simulink model "UNIFIER"  (R2023b)
settings: Solver=ode1  StartTime=0.0  StopTime=194  FixedStep=1/500  RelTol=1e-3
values from neighbouring files (symbols this model uses):
  b = 20.11467    [UNIFIERLanding_20240613_190735.mat]    (also in UNIFIER_LOAD.m; UNIFIER_LOADsim.m; UNIFIER_trim_out_20240612_032607.mat)
  c = 1.43676    [UNIFIERLanding_20240613_190735.mat]    (also in UNIFIER_LOAD.m; UNIFIER_LOADsim.m; UNIFIER_trim_out_20240612_032607.mat)
  DEP_INTEG_IC = 117.49388    [UNIFIER_LOAD.m]    (also in UNIFIER_LOADsim.m; UNIFIER_trim_out_20240612_032607.mat)
  dp_DEP =     [UNIFIERLanding_20240613_190735.mat]    (also in UNIFIER_trim_out_20240612_032607.mat)
  dp_FUSE_FIN =     [UNIFIER_trim_out_20240612_032607.mat]
  dp_HTU =     [UNIFIERLanding_20240613_190735.mat]    (also in UNIFIER_trim_out_20240612_032607.mat)
  dp_VTAIL =     [UNIFIER_trim_out_20240612_032607.mat]
  dp_VTAIL_INDUCED =     [UNIFIER_trim_out_20240612_032607.mat]
  dp_WING_root =     [UNIFIER_trim_out_20240612_032607.mat]
  dp_WING_tip =     [UNIFIER_trim_out_20240612_032607.mat]
  dumax = [1.0471975512 1.0471975512 1.0471975512 0.174532925199 2 2 2]    [UNIFIERLanding_20240613_190735.mat]
  Euler0 = xstar(7:9)'    [UNIFIER_6DOFsim_init.m]    (also in UNIFIER_LOAD.m = [0, 0, 0]; UNIFIER_LOADsim.m = [0, 0, 0]; UNIFIER_trim_out_20240612_032607.mat = [3.43106170069e-06 0.0515008506278 -2.79252663434])
  ground_alt = 0    [UNIFIER_LOAD.m]    (also in UNIFIER_LOADsim.m; UNIFIER_trim_out_20240612_032607.mat)
  m = 7057    [UNIFIERLanding_20240613_190735.mat]    (also in UNIFIER_LOAD.m; UNIFIER_LOADsim.m; UNIFIER_trim_out_20240612_032607.mat)
  omegab0 = xstar(10:12)'    [UNIFIER_6DOFsim_init.m]    (also in UNIFIER_LOAD.m = [0,0,0]; UNIFIER_LOADsim.m = [0,0,0]; UNIFIER_trim_out_20240612_032607.mat = [0 0 0])
  S = 29.98388    [UNIFIERLanding_20240613_190735.mat]    (also in UNIFIER_LOAD.m; UNIFIER_LOADsim.m; UNIFIER_trim_out_20240612_032607.mat)
  sensor_delay_steps = 5    [UNIFIER_LOAD.m]    (also in UNIFIER_LOADsim.m; UNIFIER_trim_out_20240612_032607.mat)
  solution =     [UNIFIERLanding_20240613_190735.mat]
  u1_0 = [ustar(1), -1*ustar(1), ustar(3)-ustar(2), ustar(3)+ustar(2), ustar(4), ustar(4)]    [UNIFIER_6DOFsim_init.m]    (also in UNIFIER_LOAD.m = [2.1112539e-05, -2.1112539e-05, -0.085004635, -0.084972650, ; UNIFIER_LOADsim.m = [2.1112539e-05, -2.1112539e-05, -0.085004635, -0.084972650, ; UNIFIER_trim_out_20240612_032607.mat = [2.1112539e-05 -2.1112539e-05 -0.085004635 -0.08497265 0.197)
  u2_0 = ones(1,12) .* ustar(5)    [UNIFIER_6DOFsim_init.m]    (also in UNIFIER_LOAD.m = ones(1,12) .* 0.4252; UNIFIER_LOADsim.m = ones(1,12) .* 0.4252; UNIFIER_trim_out_20240612_032607.mat = [0.4252 0.4252 0.4252 0.4252 0.4252 0.4252 0.4252 0.4252 0.4)
  u3_0 = ustar(7)    [UNIFIER_6DOFsim_init.m]    (also in UNIFIER_LOAD.m = 0.089689; UNIFIER_LOADsim.m = 0.089689; UNIFIER_trim_out_20240612_032607.mat = 0.089689)
  u4_0 = 0    [UNIFIER_6DOFsim_init.m]    (also in UNIFIER_LOAD.m; UNIFIER_LOADsim.m; UNIFIER_trim_out_20240612_032607.mat)
  u_trim = ustar    [UNIFIER_6DOFsim_init.m]    (also in UNIFIER_LOAD.m = [0.0; UNIFIER_LOADsim.m = [0.0)
  umax = [0.436332312999 0.523598775598 0.523598775598 0.436332312999 1 1 1]    [UNIFIERLanding_20240613_190735.mat]    (also in UNIFIER_trim_out_20240612_032607.mat)
  umin = [-0.436332312999 -0.523598775598 -0.523598775598 0 0 -1 -0.5]    [UNIFIERLanding_20240613_190735.mat]    (also in UNIFIER_trim_out_20240612_032607.mat)
  Va = [72.7399985115 72.2978466179 70.3592089076 68.5755686022 67.5674222915 66.8967003826 65.8958642605 64.4243196248 62.667507398 61.0171213882 59.8601734245 59.2796795419 ... (250 elements, 250x1)]    [UNIFIERLanding_20240613_190735.mat]
  Vb0 = xstar(4:6)'    [UNIFIER_6DOFsim_init.m]    (also in UNIFIER_LOAD.m = [72.731047032614440, 0, 1.142307104518741]; UNIFIER_LOADsim.m = [72.731047032614440, 0, 1.142307104518741]; UNIFIER_trim_out_20240612_032607.mat = [52.6789583502 0 2.71559652634])
  vtail_dist_to_wing = 7.8070    (= 7.807)    [UNIFIER_LOAD.m]    (also in UNIFIER_LOADsim.m; UNIFIER_trim_out_20240612_032607.mat)
  vtail_nodes = [dp_VTAIL.Xs_LE;     dp_VTAIL.Ys_LE;     dp_VTAIL.Zs_LE]    [UNIFIER_LOAD.m]    (also in UNIFIER_LOADsim.m; UNIFIER_trim_out_20240612_032607.mat = [-16.4894695282 -2.83441376686 -2.73765826225 -16.1370849609)
  wing_nodes = [fliplr(dp_WING_tip.LE_Xs),fliplr(dp_WING_root.LE_Xs),dp_WING_root.LE_Xs,dp_WING_tip.LE_Xs;     fliplr(-dp_WING_tip.LE_Ys),fliplr(-dp_WING_root.LE_Ys),dp_WING_root.LE_Ys,dp_WING_tip.LE_Ys;     fliplr(dp_WING_tip.LE_Zs),fliplr(dp_WING_root.LE_Zs),dp_WING_root.LE_Zs,dp_WING_tip.LE_Zs]    [UNIFIER_LOAD.m]    (also in UNIFIER_LOADsim.m; UNIFIER_trim_out_20240612_032607.mat = [-7.70795631409 -9.67500019073 -0.98178178072 -7.66801691055)
  Xe0 = xstar(1:3)'    [UNIFIER_6DOFsim_init.m]    (also in UNIFIER_LOAD.m = [0,0,-1219]; UNIFIER_LOADsim.m = [0,0,-1219]; UNIFIER_trim_out_20240612_032607.mat = [0 0 -1100])
  xyz_cg = [-8.09 0 -0.2]    [UNIFIERLanding_20240613_190735.mat]    (also in UNIFIER_LOAD.m = [-8.09,0,-0.2]; UNIFIER_LOADsim.m = [-8.09,0,-0.2]; UNIFIER_trim_out_20240612_032607.mat)
  xyz_DEP = [-6.9629998 -10.05 -0.90899998 -6.921 -8.4499998 -0.792 -6.8660002 -6.8499999 -0.82300001 -6.8099999 -5.25 -0.85000002 ... (36 elements, 3x12)]    [UNIFIERLanding_20240613_190735.mat]    (also in UNIFIER_LOAD.m = [ -6.9629998	-6.9210000	-6.8660002	-6.8099999	-6.7540002	-6.; UNIFIER_LOADsim.m = [ -6.9629998	-6.9210000	-6.8660002	-6.8099999	-6.7540002	-6.; UNIFIER_trim_out_20240612_032607.mat)
undefined symbols (not defined in the file or in its folder): Earth, F, MIL, WGS84
libraries: simulink_extras x23, aerolibactuator x16, dspnetwork x15, sharedutil x14, sharedtransform x7, aerolibtransform2 x5, slpidlib x5, simulink x5, aerolibwind2 x4, matrix_library x1, shared6dof x1, aerolibatmos2 x1
(part 3 of 6)

== system UNIFIER/C7A_HARW/Aero/additionalDrag ==
  note: Landing gear drag:
      | Loftin Jr, L. K. (1980). Subsonic aircraft: Evolution and the matching of size to performance (No. L-13367).
  note: Wing mounted nacelles:
      | (Estimate using OpenVSP - Jenkinson Wing Mounted Nacelle)
      | =6*0.00043=0.00258
      | + cooling drag of 0.015
  alpha (rad) : Inport
  beta (rad) : Inport  Port=2
  Vrw_mag : Inport  Port=3
  rho (kg/m^3) : Inport  Port=4
  u4 (gear) : Inport  Port=5
  Cast : DataTypeConversion  OutDataTypeStr=single  SaturateOnIntegerOverflow=off  RndMeth=Floor
  Cast1 : DataTypeConversion  OutDataTypeStr=single  SaturateOnIntegerOverflow=off  RndMeth=Floor
  Cast2 : DataTypeConversion  OutDataTypeStr=double  SaturateOnIntegerOverflow=off  RndMeth=Floor
  Constant1 : Constant  Value=0  OutDataTypeStr=single
  Direction Cosine Matrix Body to Wind : aerolibtransform2/Direction Cosine Matrix Body to Wind
  Gain : Gain  Gain=S/2
  Math Function : Math  Operator=square
  Mux : Mux  Inputs=2
  Mux1 : Mux  Inputs=3
  Product : Product  OutDataTypeStr=single
  Product1 : Product  Multiplication=Matrix(*)
  Product2 : Product
  Product3 : Product
  Sum : Sum  Inputs=|++
  Transpose : Math  Operator=transpose
  Unary Minus : UnaryMinus
  extra_drag : Constant  Value=0.00258+0.015  OutDataTypeStr=single
  gear_drag : Constant  Value=0.015  OutDataTypeStr=single
  F_additional : Outport
  wires:
  alpha (rad)/1 -> Mux/1
  Math Function/1 -> Product/2
  Product/1 -> Unary Minus/1
  Gain/1 -> Product/1
  Product2/1 -> Gain/1
  extra_drag/1 -> Sum/1
  Vrw_mag/1 -> Math Function/1
  rho (kg/m^3)/1 -> Product2/2
  Direction Cosine Matrix Body to Wind/1 -> Cast1/1
  Mux/1 -> Cast2/1
  beta (rad)/1 -> Mux/2
  Unary Minus/1 -> Mux1/1
  Transpose/1 -> Product1/1
  Mux1/1 -> Product1/2
  Constant1/1 -> Mux1/2, Mux1/3
  Product1/1 -> Cast/1
  Cast/1 -> F_additional/1
  Cast1/1 -> Transpose/1
  Cast2/1 -> Direction Cosine Matrix Body to Wind/1
  u4 (gear)/1 -> Product3/2
  gear_drag/1 -> Product3/1
  Sum/1 -> Product2/1
  Product3/1 -> Sum/2

== system UNIFIER/C7A_HARW/EOMandEnviroment1/Conversion ==
  Vrw : Inport
  rho : Inport  Port=2
  Add : Sum
  Constant1 : Constant  Value=eps
  Demux3 : Demux  Outputs=3
  Divide1 : Product  Inputs=*/
  Dot Product : DotProduct  OutDataTypeStr=Inherit: Inherit via internal rule
  Gain : Gain  Gain=1/1.225
  Product : Product
  Sqrt : Sqrt
  Sqrt1 : Sqrt
  Trigonometric Function : Trigonometry  Operator=atan2
  Trigonometric Function1 : Trigonometry  Operator=asin
  Vrw_mag : Outport
  Vrw_mag_eas : Outport  Port=2
  alpha : Outport  Port=3
  beta : Outport  Port=4
  wires:
  Demux3/2 -> Divide1/1
  Constant1/1 -> Add/2
  Sqrt/1 -> Add/1
  Divide1/1 -> Trigonometric Function1/1
  Vrw/1 -> Dot Product/1, Dot Product/2, Demux3/1  "V_w"
  Demux3/3 -> Trigonometric Function/1
  Dot Product/1 -> Sqrt/1
  Demux3/1 -> Trigonometric Function/2
  Trigonometric Function1/1 -> beta/1  "beta"
  Trigonometric Function/1 -> alpha/1  "alpha"
  rho/1 -> Gain/1
  Gain/1 -> Sqrt1/1
  Sqrt1/1 -> Product/2
  Product/1 -> Vrw_mag_eas/1
  Add/1 -> Vrw_mag/1, Product/1, Divide1/2

== system UNIFIER/C7A_HARW/EOMandEnviroment1/Enviroment ==
  Xe : Inport
  Vb : Inport  Port=2  PortDimensions=3
  DCM : Inport  Port=3
  omega : Inport  Port=4
  Cast : DataTypeConversion  OutDataTypeStr=single  SaturateOnIntegerOverflow=off  RndMeth=Floor
  Demux : Demux  Outputs=3
  ISA Atmosphere Model : aerolibatmos2/ISA Atmosphere Model  useExtended=off  action=Warning  custom=off  viscosityOut=off  g=9.80665  gamma=1.4  R=287.0531  L=0.0065  h_trop=11000  h_strat=20000  rho0=1.225  P0=101325  T0=288.15  h0=0
  Manual Switch : ManualSwitch
  Manual Switch1 : ManualSwitch  CurrentSetting=0
  Square : Math  Operator=square
  Square Root : Sqrt
  Sum : Sum  Inputs=|++
  Sum of Elements : Sum  Inputs=+
  Sum1 : Sum  Inputs=++|
  Terminator : Terminator
  Terminator1 : Terminator
  Terminator2 : Terminator
  Unary Minus : UnaryMinus
  Wind model : Subsystem
  scope_V : Subsystem
  scope_omega : Subsystem
  Vrw : Outport
  omegaw : Outport  Port=2
  T : Outport  Port=3
  P : Outport  Port=4
  rho : Outport  Port=5
  wires:
  Xe/1 -> Demux/1
  Demux/3 -> Unary Minus/1  "z"
  Demux/1 -> Terminator/1
  Demux/2 -> Terminator1/1
  ISA Atmosphere Model/2 -> Terminator2/1
  Manual Switch/1 -> Vrw/1
  Manual Switch1/1 -> omegaw/1
  Square Root/1 -> Wind model/2(Vb_mag)
  omega/1 -> scope_omega/2(<omega>), Manual Switch1/2, Sum/2
  Wind model/2(omegab_wind) -> Sum/1
  Wind model/1(Vb_wind) -> Sum1/2
  Sum1/1 -> Manual Switch/2, scope_V/1(V_w)
  Sum/1 -> scope_omega/1(omega_w), Manual Switch1/1
  ISA Atmosphere Model/1 -> T/1  "T"
  ISA Atmosphere Model/3 -> P/1  "P"
  ISA Atmosphere Model/4 -> rho/1  "rho"
  Unary Minus/1 -> Cast/1, Wind model/1(h)  "h"
  Cast/1 -> ISA Atmosphere Model/1
  DCM/1 -> Wind model/3(DCM)
  Vb/1 -> scope_V/2(<V_b>), Manual Switch/1, Sum1/1, Square/1
  Square/1 -> Sum of Elements/1
  Sum of Elements/1 -> Square Root/1

== system UNIFIER/C7A_HARW/Subsystems/Actuators ==
  u1 : Inport
  Demux : Demux  Commented=on  Outputs=6
  Mux : Mux  Commented=on  Inputs=6
  Nonlinear Second-Order Actuator : aerolibactuator/Nonlinear Second-Order Actuator  Commented=on  wn_fin=50  z_fin=0.8  fin_max=30*pi/180  fin_min=-30*pi/180  fin_maxrate=120*pi/180  fin_act_0=0  fin_act_vel=0
  Nonlinear Second-Order Actuator1 : aerolibactuator/Nonlinear Second-Order Actuator  Commented=on  wn_fin=50  z_fin=0.8  fin_max=30*pi/180  fin_min=-30*pi/180  fin_maxrate=120*pi/180  fin_act_0=0  fin_act_vel=0
  Nonlinear Second-Order Actuator2 : aerolibactuator/Nonlinear Second-Order Actuator  Commented=on  wn_fin=50  z_fin=0.8  fin_max=25*pi/180  fin_min=0  fin_maxrate=60*pi/180  fin_act_0=0  fin_act_vel=0
  Nonlinear Second-Order Actuator3 : aerolibactuator/Nonlinear Second-Order Actuator  Commented=on  wn_fin=50  z_fin=0.8  fin_max=25*pi/180  fin_min=0  fin_maxrate=60*pi/180  fin_act_0=0  fin_act_vel=0
  Nonlinear Second-Order Actuator4 : aerolibactuator/Nonlinear Second-Order Actuator  Commented=on  wn_fin=50  z_fin=0.8  fin_max=25*pi/180  fin_min=-25*pi/180  fin_maxrate=120*pi/180  fin_act_0=0  fin_act_vel=0
  Nonlinear Second-Order Actuator5 : aerolibactuator/Nonlinear Second-Order Actuator  Commented=on  wn_fin=50  z_fin=0.8  fin_max=25*pi/180  fin_min=-25*pi/180  fin_maxrate=120*pi/180  fin_act_0=0  fin_act_vel=0
  u1_actual : Outport
  wires:
  u1/1 -> u1_actual/1
  Demux/3 -> Nonlinear Second-Order Actuator/1
  Nonlinear Second-Order Actuator/1 -> Mux/3
  Demux/4 -> Nonlinear Second-Order Actuator1/1
  Nonlinear Second-Order Actuator1/1 -> Mux/4
  Demux/5 -> Nonlinear Second-Order Actuator2/1
  Demux/6 -> Nonlinear Second-Order Actuator3/1
  Nonlinear Second-Order Actuator3/1 -> Mux/6
  Nonlinear Second-Order Actuator2/1 -> Mux/5
  Demux/1 -> Nonlinear Second-Order Actuator5/1
  Nonlinear Second-Order Actuator5/1 -> Mux/1
  Nonlinear Second-Order Actuator4/1 -> Mux/2
  Demux/2 -> Nonlinear Second-Order Actuator4/1

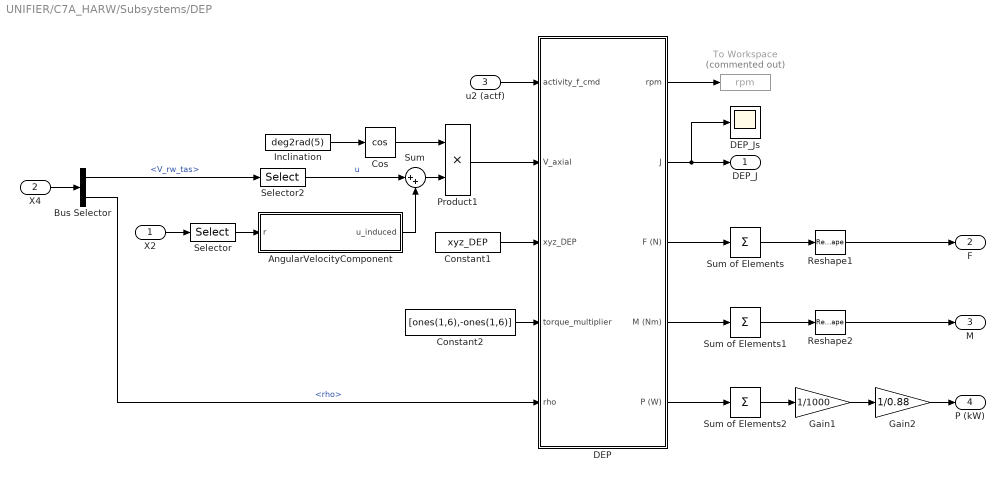
== system UNIFIER/C7A_HARW/Subsystems/DEP ==
  X2 : Inport
  X4 : Inport  Port=2
  u2 (actf) : Inport  Port=3
  AngularVelocityComponent : Subsystem
  Bus Selector : BusSelector  OutputSignals=V_rw_tas,rho
  Constant1 : Constant  Value=xyz_DEP
  Constant2 : Constant  Value=[ones(1,6),-ones(1,6)]
  Cos : Trigonometry  Operator=cos
  DEP : Subsystem  TreatAsAtomicUnit=on
  DEP_Js : Scope
  Gain1 : Gain  Gain=1/1000
  Gain2 : Gain  Gain=1/0.88
  Inclination : Constant  Value=deg2rad(5)
  Product1 : Product
  Reshape1 : Reshape
  Reshape2 : Reshape
  Selector : Selector  InputPortWidth=6  IndexOptions=Index vector (dialog)  Indices=6  OutputSizes=1
  Selector2 : Selector  InputPortWidth=3  IndexOptions=Index vector (dialog)  Indices=1  OutputSizes=1
  Sum : Sum  Inputs=|++
  Sum of Elements : Sum  Inputs=+  CollapseMode=Specified dimension  CollapseDim=2
  Sum of Elements1 : Sum  Inputs=+  CollapseMode=Specified dimension  CollapseDim=2
  Sum of Elements2 : Sum  Inputs=+  CollapseMode=Specified dimension
  To Workspace : ToWorkspace  Commented=on  VariableName=rpm  SaveFormat=Structure With Time  SampleTime=1/100
  DEP_J : Outport
  F : Outport  Port=2
  M : Outport  Port=3
  P (kW) : Outport  Port=4
  wires:
  X2/1 -> Selector/1
  X4/1 -> Bus Selector/1
  Bus Selector/1 -> Selector2/1  "<V_rw_tas>"
  Product1/1 -> DEP/2(V_axial)
  u2 (actf)/1 -> DEP/1(activity_f_cmd)
  DEP/1(rpm) -> To Workspace/1
  DEP/3(F (N)) -> Sum of Elements/1
  DEP/4(M (Nm)) -> Sum of Elements1/1
  Sum of Elements/1 -> Reshape1/1
  Sum of Elements1/1 -> Reshape2/1
  Reshape1/1 -> F/1
  Reshape2/1 -> M/1
  Constant1/1 -> DEP/3(xyz_DEP)
  Constant2/1 -> DEP/4(torque_multiplier)
  Bus Selector/2 -> DEP/5(rho)  "<rho>"
  DEP/2(J) -> DEP_Js/1, DEP_J/1
  DEP/5(P (W)) -> Sum of Elements2/1
  Sum of Elements2/1 -> Gain1/1
  Selector2/1 -> Sum/1  "u"
  Inclination/1 -> Cos/1
  Cos/1 -> Product1/1
  Sum/1 -> Product1/2
  Gain1/1 -> Gain2/1
  Gain2/1 -> P (kW)/1
  Selector/1 -> AngularVelocityComponent/1(r)
  AngularVelocityComponent/1(u_induced) -> Sum/2

== system UNIFIER/C7A_HARW/Subsystems/Gravity ==
  X4 : Inport
  Bus Selector : BusSelector  OutputSignals=DCMbe
  Constant : Constant  Value=0
  Constant1 : Constant  Value=m
  Multiply : Gain  Gain=9.80665
  Mux : Mux  Inputs=3
  Product : Product  Multiplication=Matrix(*)
  F : Outport
  wires:
  Product/1 -> F/1  "F"
  Bus Selector/1 -> Product/1  "<DCMbe>"
  X4/1 -> Bus Selector/1
  Multiply/1 -> Mux/3
  Constant/1 -> Mux/2, Mux/1
  Mux/1 -> Product/2
  Constant1/1 -> Multiply/1

== system UNIFIER/C7A_HARW/Subsystems/HTU ==
  u3 (actf) : Inport
  X4 : Inport  Port=2
  1-D Lookup Table1 : Lookup_n-D  NumberOfTableDimensions=1  BreakpointsForDimension1=[-0.5,1.5]  IndexSearchMethod=Linear search  BeginIndexSearchUsingPreviousIndexResult=on  Table=[-5000, 15000]  ExtrapMethod=Clip  InternalRulePriority=Speed  RndMeth=Simplest
  Bus Selector : BusSelector  OutputSignals=V_rw_mag_eas
  Constant : Constant  Value=0
  Gain : Gain  Gain=1/0.92
  Mux : Mux  Inputs=3
  Mux1 : Mux  Inputs=3
  PropAndMotor : Subsystem
  Scope : Scope
  To Workspace : ToWorkspace  Commented=on  VariableName=HTU  SaveFormat=Structure With Time  SampleTime=1/100
  F (N) : Outport
  M (Nm) : Outport  Port=2
  P (kW) : Outport  Port=3
  wires:
  Mux1/1 -> M (Nm)/1
  Constant/1 -> Mux1/2, Mux1/3, Mux1/1, Mux/3, Mux/2
  Mux/1 -> F (N)/1
  PropAndMotor/2(T (N)) -> Scope/1, To Workspace/1, Mux/1
  PropAndMotor/1(P (kW)) -> Gain/1
  X4/1 -> Bus Selector/1
  1-D Lookup Table1/1 -> PropAndMotor/2(T_cmd (N))
  Bus Selector/1 -> PropAndMotor/1(Vrw_mag_eas)  "<V_rw_mag_eas>"
  u3 (actf)/1 -> 1-D Lookup Table1/1
  Gain/1 -> P (kW)/1

== system UNIFIER/C7A_HARW/Subsystems/LandingGears ==
  X2 : Inport
  X3 : Inport  Port=2
  sidestick_bus : Inport  Port=3
  Constant : Constant  Value=[-8.8,-2,2]
  Constant1 : Constant  Value=[-8.8,2,2]
  Constant2 : Constant  Value=[-1.3,0,1.9]
  Constant3 : Constant  Value=ground_alt
  Demux : Demux  Outputs=2
  Demux1 : Demux  Outputs=2
  LeftMain : Subsystem
  Nose : Subsystem
  OR : Logic  Operator=OR  IconShape=distinctive  AllPortsSameDT=off  OutDataTypeStr=boolean
  RightMain : Subsystem
  Selector : Selector  InputPortWidth=3  IndexOptions=Index vector (dialog)  Indices=3  OutputSizes=1
  Selector1 : Selector  InputPortWidth=3  IndexOptions=Index vector (dialog)  Indices=3  OutputSizes=1
  SideForceAndSteeringAndBraking : Subsystem
  Sum : Sum
  Sum1 : Sum  Inputs=++++
  Sum2 : Sum  Inputs=++++
  F : Outport
  M : Outport  Port=2
  wires:
  Constant/1 -> LeftMain/1(xyz_gear)
  Constant1/1 -> RightMain/1(xyz_gear)
  Constant2/1 -> Nose/1(xyz_gear)
  X2/1 -> Demux/1
  Demux/1 -> Nose/6(V_b), RightMain/6(V_b), LeftMain/6(V_b), SideForceAndSteeringAndBraking/3(V_b)
  Demux/2 -> LeftMain/5(omega), Nose/5(omega), RightMain/5(omega)
  X3/1 -> Demux1/1
  Demux1/1 -> Nose/3(X_e), RightMain/3(X_e), LeftMain/3(X_e)
  Demux1/2 -> Nose/2(Euler), RightMain/2(Euler), LeftMain/2(Euler)
  Constant3/1 -> Nose/4(ground_alt), RightMain/4(ground_alt), LeftMain/4(ground_alt)
  Sum/1 -> Selector/1
  LeftMain/1(F) -> Sum1/2, Sum/1
  RightMain/1(F) -> Sum1/3, Sum/2
  Nose/1(F) -> Selector1/1, Sum1/4
  OR/1 -> SideForceAndSteeringAndBraking/1(impact_flag_main)
  Selector/1 -> SideForceAndSteeringAndBraking/4(Fz_main)
  Sum2/1 -> M/1
  LeftMain/3(impact_flag) -> OR/1
  RightMain/3(impact_flag) -> OR/2
  Nose/3(impact_flag) -> SideForceAndSteeringAndBraking/2(impact_flag_nose)
  sidestick_bus/1 -> SideForceAndSteeringAndBraking/6(sidestick_bus)
  SideForceAndSteeringAndBraking/1(F_b) -> Sum1/1
  LeftMain/2(M) -> Sum2/2
  RightMain/2(M) -> Sum2/3
  Nose/2(M) -> Sum2/4
  SideForceAndSteeringAndBraking/2(M_b) -> Sum2/1
  Sum1/1 -> F/1
  Selector1/1 -> SideForceAndSteeringAndBraking/5(Fz_nose)

== system UNIFIER/C7A_HARW/Subsystems/Scopes ==
  actual : Inport
  cmd : Inport  Port=2
  Demux2 : Demux  Outputs=6
  Demux3 : Demux  Outputs=6
  Mux{,1..3} (4 alike) : Mux  Inputs=2
  Radians to Degrees : simulink_extras/Transformations/Radians to Degrees
  Radians to Degrees1 : simulink_extras/Transformations/Radians to Degrees
  Surface_deflection : Scope  NumInputPorts=4
  Terminator{3..6} (4 alike) : Terminator
  wires:
  Radians to Degrees1/1 -> Demux3/1
  Demux2/2 -> Mux1/1  "aileR_actual"
  Mux2/1 -> Surface_deflection/2
  Mux1/1 -> Surface_deflection/3
  actual/1 -> Radians to Degrees/1
  Demux3/1 -> Mux/2  "aileL_cmd"
  Mux/1 -> Surface_deflection/1
  Radians to Degrees/1 -> Demux2/1
  Demux3/4 -> Mux3/1  "rudeR_cmd"
  Demux2/5 -> Terminator3/1  "flapL_actual"
  Demux2/1 -> Mux/1  "aileL_actual"
  Demux3/3 -> Mux2/2  "rudeL_cmd"
  Demux2/4 -> Mux3/2  "rudeR_actual"
  Demux3/2 -> Mux1/2  "aileR_cmd"
  Mux3/1 -> Surface_deflection/4
  Demux2/3 -> Mux2/1  "rudeL_actual"
  Demux3/6 -> Terminator6/1  "flapR_cmd"
  cmd/1 -> Radians to Degrees1/1
  Demux2/6 -> Terminator4/1  "flapR_actual"
  Demux3/5 -> Terminator5/1  "flapL_cmd"

== system UNIFIER/FCC/Ganging/For Each Subsystem ==
  zeta : Inport  Partition=on  PartitionDimension=1  PartitionWidth=1  PartitionOffset=0
  DEP_col : Inport  Port=2
  DEP_slope : Inport  Port=3
  Add : Sum
  Display : Display
  For Each : ForEach  DisableCoverage=on
  K_slope : Gain  Gain=0.785
  Product : Product
  Tan : Trigonometry  Operator=tan
  Out1 : Outport  ConcatenationDimension=1
  wires:
  DEP_slope/1 -> K_slope/1
  K_slope/1 -> Tan/1
  Tan/1 -> Product/1
  zeta/1 -> Product/2
  Product/1 -> Add/1
  DEP_col/1 -> Add/2
  Add/1 -> Display/1, Out1/1

== system UNIFIER/FCC/Ganging/V-tail mixing ==
  rud : Inport
  elev : Inport  Port=2
  Sum : Sum  Inputs=|++
  Sum1 : Sum  Inputs=|++
  Unary Minus1 : UnaryMinus
  rudL : Outport
  rudR : Outport  Port=2
  wires:
  Sum/1 -> rudL/1
  Sum1/1 -> rudR/1
  rud/1 -> Sum1/2, Unary Minus1/1
  Unary Minus1/1 -> Sum/2
  elev/1 -> Sum1/1, Sum/1

== system UNIFIER/PACER/soft real time subsystem/get elapsed wall-clock time ==
  note: Block pulled from Mathworks File Exchange entry titled " Raspberry Pi 2, get system clock with timeval "
      |
      | https://www.mathworks.com/matlabcentral/fileexchange/54546-raspberry-pi-2--get-system-clock-with-timeval
  Clock : Clock
  Compare To Zero : simulink/Logic and Bit Operations/Compare To Zero  relop===  OutDataTypeStr=boolean
  S-Function : S-Function  FunctionName=sfun_getSystemClockTimeval  SFunctionDeploymentMode=off  EnableBusSupport=off
      settings: AttributesFormatString=%<FunctionName>
  Sum : Sum  Inputs=|+-
  captured value at t==0 : Display
  elapsed wall-clock time (s) (real wall-clock seconds) : Display
  microseconds : Display
  "seconds since January 1st, 1970" : Display
  "seconds since January 1st, 1970 " : Display
  simulation seconds (s) : Display
  triggered capture & hold : Subsystem
  t_wall_clock_elapsed (s) : Outport
  wires:
  triggered capture & hold/1(out) -> captured value at t==0/1, Sum/2
  S-Function/1 -> "seconds since January 1st, 1970 "/1
  Compare To Zero/1 -> triggered capture & hold/2(trigger)
  Sum/1 -> t_wall_clock_elapsed (s)/1, elapsed wall-clock time (s) (real wall-clock seconds)/1
  S-Function/2 -> microseconds/1
  S-Function/3 -> triggered capture & hold/1(value to capture), Sum/1, "seconds since January 1st, 1970"/1
  Clock/1 -> Compare To Zero/1, simulation seconds (s)/1

== system UNIFIER/X_PLANE_VISUALS/override_flightcontrol /Subsystem ==
  value : Inport
  Constant : Constant  Value=uint8(str)
  DREF : MATLAB Function  TreatAsAtomicUnit=on
  Data Type Conversion2 : DataTypeConversion  OutDataTypeStr=single  SaturateOnIntegerOverflow=off  RndMeth=Floor
  UDP Send1 : dspnetwork/UDP Send  remoteURL='127.0.0.1'  remotePort=49000  localURL='0.0.0.0'  localPortSource=Automatically determine  localPort=-1  sendBufferSize=8192  sampletime=-1  blockPlatform=[]  separateLengthPort=0
  wires:
  Data Type Conversion2/1 -> DREF/2(value)
  DREF/1(uint8_out) -> UDP Send1/1
  Constant/1 -> DREF/1(str)
  value/1 -> Data Type Conversion2/1

== system UNIFIER/X_PLANE_VISUALS/override_flightcontrol 1/Subsystem ==
  value : Inport
  Constant : Constant  Value=uint8(str)
  DREF : MATLAB Function  TreatAsAtomicUnit=on
  Data Type Conversion2 : DataTypeConversion  OutDataTypeStr=single  SaturateOnIntegerOverflow=off  RndMeth=Floor
  UDP Send1 : dspnetwork/UDP Send  remoteURL='127.0.0.1'  remotePort=49000  localURL='0.0.0.0'  localPortSource=Automatically determine  localPort=-1  sendBufferSize=8192  sampletime=-1  blockPlatform=[]  separateLengthPort=0
  wires:
  Data Type Conversion2/1 -> DREF/2(value)
  DREF/1(uint8_out) -> UDP Send1/1
  Constant/1 -> DREF/1(str)
  value/1 -> Data Type Conversion2/1

== system UNIFIER/C7A_HARW/Aero/AlphaWIng/ComputeAlphaBetaV ==
  V_w_local : Inport
  Asin : Trigonometry  Operator=asin
  Atan : Trigonometry  Operator=atan
  Constant1 : Constant  Value=eps  OutDataTypeStr=single
  Demux : Demux  Outputs=3
  Divide : Product  Inputs=*/
  Divide1 : Product  Inputs=*/
  Dot Product : DotProduct  OutDataTypeStr=Inherit: Inherit via internal rule
  Square Root : Sqrt
  Sum2 : Sum  Inputs=|++
  alpha_nodes : Outport
  beta_nodes : Outport  Port=2
  V_nodes : Outport  Port=3
  wires:
  V_w_local/1 -> Dot Product/1, Dot Product/2, Demux/1
  Demux/2 -> Divide1/1
  Divide1/1 -> Asin/1
  Demux/1 -> Sum2/1  "u"
  Sum2/1 -> Divide/2
  Square Root/1 -> V_nodes/1, Divide1/2
  Divide/1 -> Atan/1
  Demux/3 -> Divide/1  "w"
  Asin/1 -> beta_nodes/1  "beta"
  Constant1/1 -> Sum2/2
  Dot Product/1 -> Square Root/1
  Atan/1 -> alpha_nodes/1

== system UNIFIER/C7A_HARW/Aero/FinFuselageForces/Subsystem1 ==
  beta : Inport
  alpha : Inport  Port=2
  Constant : Constant  Value=0  OutDataTypeStr=single
  Interpolation Using Prelookup : Interpolation_n-D  Table=dp_FUSE_FIN.CD  InternalRulePriority=Speed  TableDataTypeStr=single
  Interpolation Using Prelookup1 : Interpolation_n-D  Table=dp_FUSE_FIN.CS  InternalRulePriority=Speed
  Interpolation Using Prelookup3 : Interpolation_n-D  Table=dp_FUSE_FIN.CMx  InternalRulePriority=Speed
  Interpolation Using Prelookup4 : Interpolation_n-D  Table=dp_FUSE_FIN.CMy  InternalRulePriority=Speed
  Interpolation Using Prelookup5 : Interpolation_n-D  Table=dp_FUSE_FIN.CMz  InternalRulePriority=Speed
  Subsystem : Subsystem
  Cd : Outport
  Cs : Outport  Port=2
  Cl : Outport  Port=3
  CMx : Outport  Port=4
  CMy : Outport  Port=5
  CMz : Outport  Port=6
  wires:
  Interpolation Using Prelookup3/1 -> CMx/1
  Interpolation Using Prelookup/1 -> Cd/1
  Constant/1 -> Cl/1
  Interpolation Using Prelookup5/1 -> CMz/1
  beta/1 -> Subsystem/1(beta)
  Subsystem/3(Out3) -> Interpolation Using Prelookup/3, Interpolation Using Prelookup1/3, Interpolation Using Prelookup3/3, Interpolation Using Prelookup4/3, Interpolation Using Prelookup5/3
  Interpolation Using Prelookup4/1 -> CMy/1
  alpha/1 -> Subsystem/2(alpha)
  Interpolation Using Prelookup1/1 -> Cs/1
  Subsystem/4(Out4) -> Interpolation Using Prelookup/4, Interpolation Using Prelookup1/4, Interpolation Using Prelookup3/4, Interpolation Using Prelookup4/4, Interpolation Using Prelookup5/4
  Subsystem/1(Out1) -> Interpolation Using Prelookup/1, Interpolation Using Prelookup1/1, Interpolation Using Prelookup3/1, Interpolation Using Prelookup4/1, Interpolation Using Prelookup5/1
  Subsystem/2(Out2) -> Interpolation Using Prelookup/2, Interpolation Using Prelookup1/2, Interpolation Using Prelookup3/2, Interpolation Using Prelookup4/2, Interpolation Using Prelookup5/2

== system UNIFIER/C7A_HARW/Aero/InducedAngleOfAttack/addDelay ==
  V_induced : Inport
  alpha_induced : Inport  Port=2
  vtail_V_nodes : Inport  Port=3
  Cast{,1..3} (4 alike) : DataTypeConversion  OutDataTypeStr=double  SaturateOnIntegerOverflow=off  RndMeth=Floor
  Cast4 : DataTypeConversion  OutDataTypeStr=single  SaturateOnIntegerOverflow=off  RndMeth=Floor
  Cast5 : DataTypeConversion  OutDataTypeStr=single  SaturateOnIntegerOverflow=off  RndMeth=Floor
  Constant2 : Constant  Value=vtail_dist_to_wing
  Divide : Product  Inputs=*/
  Saturation : Saturate  UpperLimit=inf  LowerLimit=10
  Step : Step  SampleTime=0
  Step1 : Step  SampleTime=0
  Sum : Sum  Inputs=|++
  Switch : Switch  Criteria=u2 > Threshold  SaturateOnIntegerOverflow=off  InputSameDT=off
  Switch1 : Switch  Criteria=u2 > Threshold  SaturateOnIntegerOverflow=off  InputSameDT=off
  Variable Transport Delay : VariableTransportDelay  MaximumDelay=10  MaximumPoints=5072  ZeroDelay=on  TransDelayFeedthrough=on
  Variable Transport Delay1 : VariableTransportDelay  MaximumDelay=10  MaximumPoints=5072  ZeroDelay=on  TransDelayFeedthrough=on
  V_delayed : Outport
  alpha_delayed : Outport  Port=2
  wires:
  V_induced/1 -> Sum/1, Cast1/1
  Divide/1 -> Cast/1, Cast3/1
  Switch/1 -> Cast4/1
  Constant2/1 -> Divide/1
  alpha_induced/1 -> Cast2/1
  Switch1/1 -> Cast5/1
  Sum/1 -> Saturation/1
  vtail_V_nodes/1 -> Sum/2
  Saturation/1 -> Divide/2
  Cast1/1 -> Switch/3, Variable Transport Delay1/1
  Cast3/1 -> Variable Transport Delay/2
  Cast4/1 -> V_delayed/1
  Cast5/1 -> alpha_delayed/1
  Cast/1 -> Variable Transport Delay1/2
  Variable Transport Delay1/1 -> Switch/1
  Step/1 -> Switch/2
  Variable Transport Delay/1 -> Switch1/1
  Step1/1 -> Switch1/2
  Cast2/1 -> Switch1/3, Variable Transport Delay/1

== system UNIFIER/C7A_HARW/Aero/InducedAngleOfAttack/preLook ==
  wing_flap_defl : Inport
  wing_alphas : Inport  Port=2
  wing_V_inf : Inport  Port=3
  wing_DEP_J : Inport  Port=4
  Constant8 : Constant  Value=0:15
  Prelookup : PreLookup  BreakpointsData=dp_VTAIL_INDUCED.flap_defl  IndexSearchMethod=Linear search  BeginIndexSearchUsingPreviousIndexResult=on  ExtrapMethod=Linear
  Prelookup1 : PreLookup  BreakpointsData=dp_VTAIL_INDUCED.V_infs  IndexSearchMethod=Linear search  BeginIndexSearchUsingPreviousIndexResult=on  ExtrapMethod=Linear
  Prelookup2 : PreLookup  BreakpointsData=dp_VTAIL_INDUCED.alphas  IndexSearchMethod=Linear search  BeginIndexSearchUsingPreviousIndexResult=on  ExtrapMethod=Linear
  Prelookup3 : PreLookup  BreakpointsData=dp_VTAIL_INDUCED.DEP_J  IndexSearchMethod=Linear search  BeginIndexSearchUsingPreviousIndexResult=on
  Out1 : Outport
  Out2 : Outport  Port=2
  Out8 : Outport  Port=3
  Out9 : Outport  Port=4
  Out3 : Outport  Port=5
  Out4 : Outport  Port=6
  Out6 : Outport  Port=7
  Out7 : Outport  Port=8
  Out5 : Outport  Port=9
  wires:
  Prelookup/1 -> Out1/1
  Constant8/1 -> Out5/1
  Prelookup1/2 -> Out4/1
  Prelookup/2 -> Out2/1
  wing_V_inf/1 -> Prelookup1/1
  Prelookup1/1 -> Out3/1
  wing_flap_defl/1 -> Prelookup/1
  wing_alphas/1 -> Prelookup2/1
  wing_DEP_J/1 -> Prelookup3/1
  Prelookup3/1 -> Out6/1
  Prelookup3/2 -> Out7/1
  Prelookup2/1 -> Out8/1
  Prelookup2/2 -> Out9/1

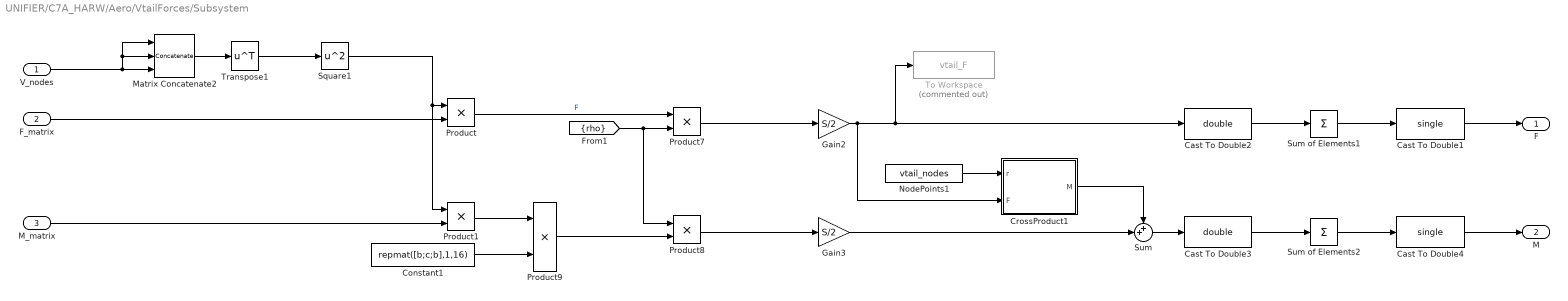
== system UNIFIER/C7A_HARW/Aero/VtailForces/Subsystem ==
  V_nodes : Inport
  F_matrix : Inport  Port=2
  M_matrix : Inport  Port=3
  Cast To Double1 : DataTypeConversion  OutDataTypeStr=single  SaturateOnIntegerOverflow=off  RndMeth=Floor
  Cast To Double2 : DataTypeConversion  OutDataTypeStr=double  SaturateOnIntegerOverflow=off  RndMeth=Floor
  Cast To Double3 : DataTypeConversion  OutDataTypeStr=double  SaturateOnIntegerOverflow=off  RndMeth=Floor
  Cast To Double4 : DataTypeConversion  OutDataTypeStr=single  SaturateOnIntegerOverflow=off  RndMeth=Floor
  Constant1 : Constant  Value=repmat([b;c;b],1,16)  VectorParams1D=off  OutDataTypeStr=single
  CrossProduct1 : Subsystem  TreatAsAtomicUnit=on
  Gain2 : Gain  Gain=S/2
  Gain3 : Gain  Gain=S/2
  Matrix Concatenate2 : Concatenate  NumInputs=3  Mode=Multidimensional array  ConcatenateDimension=2
  NodePoints1 : Constant  Value=vtail_nodes
  Product{,1,7..9} (5 alike) : Product
  Square1 : Math  Operator=square
  Sum : Sum  Inputs=++|
  Sum of Elements1 : Sum  Inputs=+  CollapseMode=Specified dimension  CollapseDim=2
  Sum of Elements2 : Sum  Inputs=+  CollapseMode=Specified dimension  CollapseDim=2
  To Workspace : ToWorkspace  Commented=on  VariableName=vtail_F  SaveFormat=Structure With Time  SampleTime=1/100
  Transpose1 : Math  Operator=transpose
  F : Outport
  M : Outport  Port=2
  wires:
  Sum/1 -> Cast To Double3/1
  Sum of Elements2/1 -> Cast To Double4/1
  Sum of Elements1/1 -> Cast To Double1/1
  Transpose1/1 -> Square1/1
  Product/1 -> Product7/1  "F"
  Product7/1 -> Gain2/1
  Square1/1 -> Product1/1, Product/1
  Matrix Concatenate2/1 -> Transpose1/1
  Gain3/1 -> Sum/2
  Product9/1 -> Product8/2
  NodePoints1/1 -> CrossProduct1/1(r)
  [rho] -> Product8/1, Product7/2
  Product8/1 -> Gain3/1
  Constant1/1 -> Product9/2
  M_matrix/1 -> Product1/2
  Product1/1 -> Product9/1
  CrossProduct1/1(M) -> Sum/1
  F_matrix/1 -> Product/2
  V_nodes/1 -> Matrix Concatenate2/1, Matrix Concatenate2/2, Matrix Concatenate2/3
  Cast To Double2/1 -> Sum of Elements1/1
  Cast To Double1/1 -> F/1
  Cast To Double3/1 -> Sum of Elements2/1
  Cast To Double4/1 -> M/1
  Gain2/1 -> CrossProduct1/2(F), To Workspace/1, Cast To Double2/1

== system UNIFIER/C7A_HARW/Aero/VtailForces/VtailForces ==
  rude_defl_nodes : Inport
  alpha_nodes : Inport  Port=2
  beta_nodes : Inport  Port=3
  Interpolation Using Prelookup1 : Interpolation_n-D  NumberOfTableDimensions=4  Table=dp_VTAIL.CFx  NumSelectionDims=1  InternalRulePriority=Speed  TableDataTypeStr=Inherit: Inherit from 'Table data'
      settings: InputPortMap=u0,u1,u2,u3,u4,u5,u6
  Interpolation Using Prelookup2 : Interpolation_n-D  NumberOfTableDimensions=4  Table=dp_VTAIL.CFy  NumSelectionDims=1  InternalRulePriority=Speed  TableDataTypeStr=Inherit: Inherit from 'Table data'
      settings: InputPortMap=u0,u1,u2,u3,u4,u5,u6
  Interpolation Using Prelookup3 : Interpolation_n-D  NumberOfTableDimensions=4  Table=dp_VTAIL.CFz  NumSelectionDims=1  InternalRulePriority=Speed  TableDataTypeStr=Inherit: Inherit from 'Table data'
      settings: InputPortMap=u0,u1,u2,u3,u4,u5,u6
  Interpolation Using Prelookup4 : Interpolation_n-D  NumberOfTableDimensions=4  Table=dp_VTAIL.CMx  NumSelectionDims=1  InternalRulePriority=Speed  TableDataTypeStr=Inherit: Inherit from 'Table data'
      settings: InputPortMap=u0,u1,u2,u3,u4,u5,u6
  Interpolation Using Prelookup5 : Interpolation_n-D  NumberOfTableDimensions=4  Table=dp_VTAIL.CMy  NumSelectionDims=1  InternalRulePriority=Speed  TableDataTypeStr=Inherit: Inherit from 'Table data'
      settings: InputPortMap=u0,u1,u2,u3,u4,u5,u6
  Interpolation Using Prelookup6 : Interpolation_n-D  NumberOfTableDimensions=4  Table=dp_VTAIL.CMz  NumSelectionDims=1  InternalRulePriority=Speed  TableDataTypeStr=Inherit: Inherit from 'Table data'
      settings: InputPortMap=u0,u1,u2,u3,u4,u5,u6
  WingRootPreLookup : Subsystem
  Cx : Outport
  Cy : Outport  Port=2
  Cz : Outport  Port=3
  CMx : Outport  Port=4
  CMy : Outport  Port=5
  CMz : Outport  Port=6
  wires:
  WingRootPreLookup/3(Out3) -> Interpolation Using Prelookup2/3, Interpolation Using Prelookup6/3, Interpolation Using Prelookup5/3, Interpolation Using Prelookup4/3, Interpolation Using Prelookup3/3, Interpolation Using Prelookup1/3
  rude_defl_nodes/1 -> WingRootPreLookup/1(rude_defl_nodes)
  WingRootPreLookup/4(Out4) -> Interpolation Using Prelookup6/4, Interpolation Using Prelookup5/4, Interpolation Using Prelookup4/4, Interpolation Using Prelookup3/4, Interpolation Using Prelookup2/4, Interpolation Using Prelookup1/4
  WingRootPreLookup/5(Out6) -> Interpolation Using Prelookup4/5, Interpolation Using Prelookup6/5, Interpolation Using Prelookup5/5, Interpolation Using Prelookup3/5, Interpolation Using Prelookup2/5, Interpolation Using Prelookup1/5
  Interpolation Using Prelookup1/1 -> Cx/1
  WingRootPreLookup/6(Out7) -> Interpolation Using Prelookup6/6, Interpolation Using Prelookup5/6, Interpolation Using Prelookup4/6, Interpolation Using Prelookup3/6, Interpolation Using Prelookup2/6, Interpolation Using Prelookup1/6
  WingRootPreLookup/2(Out2) -> Interpolation Using Prelookup4/2, Interpolation Using Prelookup5/2, Interpolation Using Prelookup6/2, Interpolation Using Prelookup3/2, Interpolation Using Prelookup2/2, Interpolation Using Prelookup1/2
  beta_nodes/1 -> WingRootPreLookup/3(beta_nodes)
  alpha_nodes/1 -> WingRootPreLookup/2(alpha_nodes)
  WingRootPreLookup/7(Out5) -> Interpolation Using Prelookup5/7, Interpolation Using Prelookup6/7, Interpolation Using Prelookup4/7, Interpolation Using Prelookup3/7, Interpolation Using Prelookup2/7, Interpolation Using Prelookup1/7
  Interpolation Using Prelookup2/1 -> Cy/1
  Interpolation Using Prelookup3/1 -> Cz/1
  Interpolation Using Prelookup4/1 -> CMx/1
  Interpolation Using Prelookup5/1 -> CMy/1
  Interpolation Using Prelookup6/1 -> CMz/1
  WingRootPreLookup/1(Out1) -> Interpolation Using Prelookup6/1, Interpolation Using Prelookup5/1, Interpolation Using Prelookup4/1, Interpolation Using Prelookup3/1, Interpolation Using Prelookup2/1, Interpolation Using Prelookup1/1

== system UNIFIER/C7A_HARW/Aero/WingForces/Left ==
  flap_defl : Inport
  aile_defl : Inport  Port=2
  DEP_J : Inport  Port=3  PortDimensions=6
  alpha : Inport  Port=4  PortDimensions=7
  V_node : Inport  Port=5  PortDimensions=7
  Matrix Concatenate1 : Concatenate  NumInputs=3  Mode=Multidimensional array  ConcatenateDimension=2
  Matrix Concatenate2 : Concatenate  NumInputs=3  Mode=Multidimensional array  ConcatenateDimension=2
  Selector : Selector  InputPortWidth=6  IndexOptions=Index vector (dialog)  Indices=[1,2,3,4,5]  OutputSizes=1
  Selector1 : Selector  InputPortWidth=6  IndexOptions=Index vector (dialog)  Indices=[5,6]  OutputSizes=1
  Selector2 : Selector  InputPortWidth=7  IndexOptions=Index vector (dialog)  Indices=[1,2,3,4,5]  OutputSizes=1
  Selector3 : Selector  InputPortWidth=7  IndexOptions=Index vector (dialog)  Indices=[6,7]  OutputSizes=1
  Selector4 : Selector  InputPortWidth=7  IndexOptions=Index vector (dialog)  Indices=[6,7]  OutputSizes=1
  Selector5 : Selector  InputPortWidth=7  IndexOptions=Index vector (dialog)  Indices=[1,2,3,4,5]  OutputSizes=1
  Subsystem : Subsystem
  Transpose : Math  Operator=transpose
  Transpose1 : Math  Operator=transpose
  Vector Concatenate{,1..5} (6 alike) : Concatenate
  WingRootForces : Subsystem
  WingTipForces : Subsystem
  F : Outport
  M : Outport  Port=2
  wires:
  flap_defl/1 -> WingRootForces/1(flap_defl)
  alpha/1 -> Subsystem/1(alpha_nodes), Selector2/1, Selector3/1
  DEP_J/1 -> Selector1/1, Selector/1
  Selector/1 -> WingRootForces/4(DEP_J)
  V_node/1 -> Selector4/1, Subsystem/2(V_nodes), Selector5/1
  WingRootForces/1(CD) -> Vector Concatenate/1
  Selector1/1 -> WingTipForces/4(DEP_J)
  WingRootForces/6(CMz) -> Vector Concatenate5/1
  WingTipForces/1(CD) -> Vector Concatenate/2
  WingTipForces/6(CMz) -> Vector Concatenate5/2
  WingTipForces/2(CS) -> Vector Concatenate1/2
  WingTipForces/3(CL) -> Vector Concatenate2/2
  WingTipForces/5(CMy) -> Vector Concatenate4/2
  WingTipForces/4(CMx) -> Vector Concatenate3/2
  aile_defl/1 -> WingTipForces/1(ail_defl)
  Selector2/1 -> WingRootForces/2(alpha)
  Selector3/1 -> WingTipForces/2(alpha)
  Selector4/1 -> WingTipForces/3(V_node)
  Selector5/1 -> WingRootForces/3(V_node)
  WingRootForces/2(CS) -> Vector Concatenate1/1
  WingRootForces/3(CL) -> Vector Concatenate2/1
  WingRootForces/4(CMx) -> Vector Concatenate3/1
  WingRootForces/5(CMy) -> Vector Concatenate4/1
  Vector Concatenate1/1 -> Matrix Concatenate1/2  "CS"
  Matrix Concatenate1/1 -> Transpose/1
  Vector Concatenate/1 -> Matrix Concatenate1/1  "CD"
  Vector Concatenate2/1 -> Matrix Concatenate1/3  "CL"
  Vector Concatenate3/1 -> Matrix Concatenate2/1  "CMx"
  Vector Concatenate4/1 -> Matrix Concatenate2/2  "CMy"
  Vector Concatenate5/1 -> Matrix Concatenate2/3  "CMz"
  Matrix Concatenate2/1 -> Transpose1/1
  Transpose/1 -> Subsystem/3(F_matrix)
  Transpose1/1 -> Subsystem/4(M_matrix)
  Subsystem/1(F) -> F/1
  Subsystem/2(M) -> M/1

== system UNIFIER/C7A_HARW/Aero/WingForces/Right ==
  flap_defl : Inport
  aile_defl : Inport  Port=2
  DEP_J : Inport  Port=3  PortDimensions=6
  alpha : Inport  Port=4  PortDimensions=7
  V_node : Inport  Port=5  PortDimensions=7
  Matrix Concatenate1 : Concatenate  NumInputs=3  Mode=Multidimensional array  ConcatenateDimension=2
  Matrix Concatenate2 : Concatenate  NumInputs=3  Mode=Multidimensional array  ConcatenateDimension=2
  Selector : Selector  InputPortWidth=6  IndexOptions=Index vector (dialog)  Indices=[1,2,3,4,5]  OutputSizes=1
  Selector1 : Selector  InputPortWidth=6  IndexOptions=Index vector (dialog)  Indices=[5,6]  OutputSizes=1
  Selector2 : Selector  InputPortWidth=7  IndexOptions=Index vector (dialog)  Indices=[1,2,3,4,5]  OutputSizes=1
  Selector3 : Selector  InputPortWidth=7  IndexOptions=Index vector (dialog)  Indices=[6,7]  OutputSizes=1
  Selector4 : Selector  InputPortWidth=7  IndexOptions=Index vector (dialog)  Indices=[6,7]  OutputSizes=1
  Selector5 : Selector  InputPortWidth=7  IndexOptions=Index vector (dialog)  Indices=[1,2,3,4,5]  OutputSizes=1
  Subsystem : Subsystem
  Transpose : Math  Operator=transpose
  Transpose1 : Math  Operator=transpose
  Vector Concatenate{,1..5} (6 alike) : Concatenate
  WingRootForces : Subsystem
  WingTipForces : Subsystem
  F : Outport
  M : Outport  Port=2
  wires:
  flap_defl/1 -> WingRootForces/1(flap_defl)
  alpha/1 -> Subsystem/1(alpha_nodes), Selector2/1, Selector3/1
  DEP_J/1 -> Selector1/1, Selector/1
  Selector/1 -> WingRootForces/4(DEP_J)
  V_node/1 -> Selector4/1, Subsystem/2(V_nodes), Selector5/1
  WingRootForces/1(CD) -> Vector Concatenate/1
  Selector1/1 -> WingTipForces/4(DEP_J)
  WingRootForces/6(CMz) -> Vector Concatenate5/1
  WingTipForces/1(CD) -> Vector Concatenate/2
  WingTipForces/6(CMz) -> Vector Concatenate5/2
  WingTipForces/2(CS) -> Vector Concatenate1/2
  WingTipForces/3(CL) -> Vector Concatenate2/2
  WingTipForces/5(CMy) -> Vector Concatenate4/2
  WingTipForces/4(CMx) -> Vector Concatenate3/2
  aile_defl/1 -> WingTipForces/1(ail_defl)
  Selector2/1 -> WingRootForces/2(alpha)
  Selector3/1 -> WingTipForces/2(alpha)
  Selector4/1 -> WingTipForces/3(V_node)
  Selector5/1 -> WingRootForces/3(V_node)
  WingRootForces/2(CS) -> Vector Concatenate1/1
  WingRootForces/3(CL) -> Vector Concatenate2/1
  WingRootForces/4(CMx) -> Vector Concatenate3/1
  WingRootForces/5(CMy) -> Vector Concatenate4/1
  Vector Concatenate1/1 -> Matrix Concatenate1/2  "CS"
  Matrix Concatenate1/1 -> Transpose/1
  Vector Concatenate/1 -> Matrix Concatenate1/1  "CD"
  Vector Concatenate2/1 -> Matrix Concatenate1/3  "CL"
  Vector Concatenate3/1 -> Matrix Concatenate2/1  "CMx"
  Vector Concatenate4/1 -> Matrix Concatenate2/2  "CMy"
  Vector Concatenate5/1 -> Matrix Concatenate2/3  "CMz"
  Matrix Concatenate2/1 -> Transpose1/1
  Transpose/1 -> Subsystem/3(F_matrix)
  Transpose1/1 -> Subsystem/4(M_matrix)
  Subsystem/1(F) -> F/1
  Subsystem/2(M) -> M/1

== system UNIFIER/C7A_HARW/Aero/WingForces/Subsystem ==
  DEP_J : Inport
  alpha_nodes : Inport  Port=2
  V_nodes : Inport  Port=3
  Demux1 : Demux  Outputs=2
  Demux2 : Demux  Outputs=2
  Demux3 : Demux  Outputs=2
  Selector : Selector  InputPortWidth=6  IndexOptions=Index vector (dialog)  Indices=[6,5,4,3,2,1]  OutputSizes=1
  Selector1 : Selector  InputPortWidth=7  IndexOptions=Index vector (dialog)  Indices=[7,6,5,4,3,2,1]  OutputSizes=1
  Selector2 : Selector  InputPortWidth=7  IndexOptions=Index vector (dialog)  Indices=[7,6,5,4,3,2,1]  OutputSizes=1
  DEP_J_Left : Outport  PortDimensions=6
  alpha_nodes_Left : Outport  Port=2  PortDimensions=7
  V_nodes_Left : Outport  Port=3  PortDimensions=7
  DEP_J_Right : Outport  Port=4  PortDimensions=6
  alpha_nodes_Right : Outport  Port=5  PortDimensions=7
  V_nodes_Right : Outport  Port=6  PortDimensions=7
  wires:
  Demux2/2 -> DEP_J_Right/1
  Demux2/1 -> Selector/1
  DEP_J/1 -> Demux2/1
  Selector/1 -> DEP_J_Left/1
  Selector1/1 -> alpha_nodes_Left/1
  alpha_nodes/1 -> Demux1/1
  Demux1/2 -> alpha_nodes_Right/1
  Demux1/1 -> Selector1/1
  Demux3/1 -> Selector2/1
  Selector2/1 -> V_nodes_Left/1
  V_nodes/1 -> Demux3/1
  Demux3/2 -> V_nodes_Right/1

== system UNIFIER/C7A_HARW/EOMandEnviroment1/Enviroment/Wind model ==
  h : Inport
  Vb_mag : Inport  Port=2
  DCM : Inport  Port=3
  Constant : Constant  Value=[0,0,0]
  Constant1 : Constant  Commented=on  Value=0.25
  Discrete Wind Gust Model : aerolibwind2/Discrete Wind Gust Model  Commented=on  units=Metric (MKS)  Gx=on  Gy=on  Gz=on  t_0=5  d_m=[120 120 80]  v_m=[3.5 3.5 3.0]
  Discrete Wind Gust Model1 : aerolibwind2/Discrete Wind Gust Model  units=Metric (MKS)  Gx=off  Gy=on  Gz=off  t_0=20  d_m=[150 150 150]  v_m=[7.71667 7.71667 7.71667]
  Dryden Wind Turbulence Model (Continuous (+q +r)) : aerolibwind2/Dryden Wind Turbulence Model  (Continuous (+q -r))  Commented=on  units=Metric (MKS)  spec=MIL-F-8785C  model=Continuous Dryden (+q +r)  W20=3  Wdeg=0  TurbProb=10^-1  L_high=533.4  Wingspan=b  ts=0.1  Seed=[23341 23342 23343 23344]  T_on=on
  Horizontal Wind Model : aerolibwind2/Horizontal Wind Model  Commented=on  units=Metric (MKS)  Vw_source=External  Vwind=15  W_source=Internal  Wdeg=245
  Integrator : Integrator  Commented=on  LimitOutput=on  UpperSaturationLimit=15  LowerSaturationLimit=0
  Scope : Scope
  Scope1 : Scope
  Terminator : Terminator
  Terminator1 : Terminator
  Vb_wind : Outport
  omegab_wind : Outport  Port=2
  wires:
  h/1 -> Dryden Wind Turbulence Model (Continuous (+q +r))/1
  Vb_mag/1 -> Discrete Wind Gust Model1/1, Dryden Wind Turbulence Model (Continuous (+q +r))/2
  DCM/1 -> Horizontal Wind Model/1, Dryden Wind Turbulence Model (Continuous (+q +r))/3
  Dryden Wind Turbulence Model (Continuous (+q +r))/1 -> Scope/1
  Dryden Wind Turbulence Model (Continuous (+q +r))/2 -> Terminator/1, Scope1/1
  Constant/1 -> omegab_wind/1
  Horizontal Wind Model/1 -> Terminator1/1
  Constant1/1 -> Integrator/1
  Integrator/1 -> Horizontal Wind Model/2
  Discrete Wind Gust Model1/1 -> Vb_wind/1

== system UNIFIER/C7A_HARW/EOMandEnviroment1/Enviroment/scope_V ==
  V_w : Inport
  <V_b> : Inport  Port=2
  Demux : Demux  Outputs=3
  Demux1 : Demux  Outputs=3
  Mux : Mux  Inputs=2
  Mux1 : Mux  Inputs=2
  Mux2 : Mux  Inputs=2
  V_comparison : Scope  NumInputPorts=3
  wires:
  V_w/1 -> Demux/1
  <V_b>/1 -> Demux1/1
  Demux/1 -> Mux/1  "w_u"
  Demux1/1 -> Mux/2  "b_u"
  Demux/2 -> Mux1/1  "w_v"
  Demux1/2 -> Mux1/2  "b_v"
  Demux/3 -> Mux2/1  "w_w"
  Demux1/3 -> Mux2/2  "b_w"
  Mux/1 -> V_comparison/1
  Mux1/1 -> V_comparison/2
  Mux2/1 -> V_comparison/3

== system UNIFIER/C7A_HARW/EOMandEnviroment1/Enviroment/scope_omega ==
  omega_w : Inport
  <omega> : Inport  Port=2
  Demux : Demux  Outputs=3
  Demux1 : Demux  Outputs=3
  Mux : Mux  Inputs=2
  Mux1 : Mux  Inputs=2
  Mux2 : Mux  Inputs=2
  omega_comparison : Scope  NumInputPorts=3
  wires:
  omega_w/1 -> Demux/1
  <omega>/1 -> Demux1/1
  Demux/1 -> Mux/1  "w_p"
  Demux1/1 -> Mux/2  "b_p"
  Demux/2 -> Mux1/1  "w_q"
  Demux1/2 -> Mux1/2  "b_q"
  Demux/3 -> Mux2/1  "w_r"
  Demux1/3 -> Mux2/2  "b_r"
  Mux/1 -> omega_comparison/1
  Mux1/1 -> omega_comparison/2
  Mux2/1 -> omega_comparison/3

== system UNIFIER/C7A_HARW/Subsystems/DEP/AngularVelocityComponent ==
  r : Inport
  Constant : Constant  Value=xyz_DEP
  Constant4 : Constant  Value=xyz_cg
  Gain : Gain  Gain=ones(1,12)
  Product : Product
  Reshape : Reshape
  Reshape3 : Reshape
  Selector1 : Selector  NumberOfDimensions=2  InputPortWidth=6  IndexOptions=Index vector (dialog),Select all  Indices=2,1  OutputSizes=1,1
  Selector3 : Selector  InputPortWidth=3  IndexOptions=Index vector (dialog)  Indices=2  OutputSizes=1
  Sum1 : Sum  Inputs=|+-
  u_induced : Outport
  wires:
  Selector1/1 -> Reshape/1
  Constant4/1 -> Selector3/1
  Sum1/1 -> Product/2
  Selector3/1 -> Gain/1
  Gain/1 -> Reshape3/1
  Reshape3/1 -> Sum1/1
  r/1 -> Product/1
  Constant/1 -> Selector1/1
  Reshape/1 -> Sum1/2
  Product/1 -> u_induced/1
